simulink model "Lab2 "  (R2019a)
settings: Solver=VariableStepAuto  StartTime=0.0  StopTime=1000  RelTol=1e-3
settings Model: Creator=jiahua  LastModifiedBy=jiahua

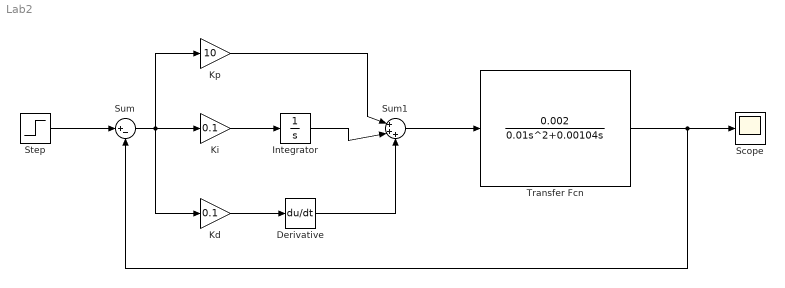
== system Lab2  ==
  Derivative : Derivative
  Integrator : Integrator
  Kd : Gain  Gain=0.1
  Ki : Gain  Gain=0.1
  Kp : Gain  Gain=10
  Scope : Scope
  Step : Step  SampleTime=0
  Sum : Sum  Inputs=|+-
  Sum1 : Sum  Inputs=|+++
  Transfer Fcn : TransferFcn  Numerator=[0.002]  Denominator=[0.01,0.00104,0]
  wires:
  Transfer Fcn/1 -> Sum/2, Scope/1
  Step/1 -> Sum/1
  Sum/1 -> Kd/1, Ki/1, Kp/1
  Kp/1 -> Sum1/1
  Kd/1 -> Derivative/1
  Derivative/1 -> Sum1/3
  Ki/1 -> Integrator/1
  Integrator/1 -> Sum1/2
  Sum1/1 -> Transfer Fcn/1
